simulink model "induction_machine_PeiXu_5186611"  (Simulink 8.6)
settings: Solver=ode45  StartTime=0  StopTime=25  RelTol=1e-3
libraries: aerolibutil x8
settings Model: Creator=XP  LastModifiedBy=XP
settings DataIOCC: SignalLoggingSaveFormat=Dataset
settings OptimizationCC: ExpressionDepthLimit=128
settings DebuggingCC: UnderspecifiedInitializationDetection=Simplified  MergeDetectMultiDrivingBlocksExec=error  FcnCallInpInsideContextMsg=EnableAllAsError  StateNameClashWarn=none
settings GRTTargetCC: CombineOutputUpdateFcns=on  GRTInterface=off
settings ConfigComp: CovSFcnEnable=off

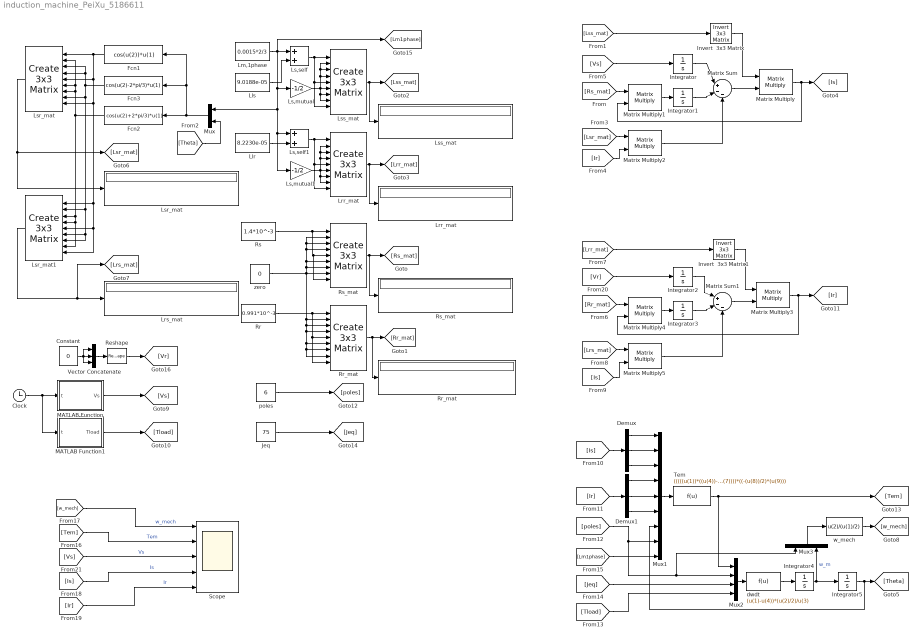
== system induction_machine_PeiXu_5186611 ==
  Clock : Clock
  Constant : Constant  Value=0
  Demux : Demux  Outputs=3
  Demux1 : Demux  Outputs=3
  Fcn1 : Fcn  Expr=cos(u(2))*u(1)
  Fcn2 : Fcn  Expr=cos(u(2)+2*pi/3)*u(1)
  Fcn3 : Fcn  Expr=cos(u(2)-2*pi/3)*u(1)
  Integrator{,1..5} (6 alike) : Integrator
  Invert  3x3 Matrix : aerolibutil/Invert  3x3 Matrix
  Invert  3x3 Matrix1 : aerolibutil/Invert  3x3 Matrix
  Jeq : Constant  Value=75
  Llr : Constant  Value=8.2230e-05
  Lls : Constant  Value=9.0188e-05
  Lm,1phase : Constant  Value=0.0015*2/3
  Lrr_mat : aerolibutil/Create 3x3 Matrix
  "Lrr_mat " : Display
  "Lrs_mat " : Display
  Ls,mutual : Gain  Gain=-1/2
  Ls,mutual1 : Gain  Gain=-1/2
  Ls,self : Sum
  Ls,self1 : Sum
  Lsr_mat : aerolibutil/Create 3x3 Matrix
  "Lsr_mat " : Display
  Lsr_mat1 : aerolibutil/Create 3x3 Matrix
  Lss_mat : aerolibutil/Create 3x3 Matrix
  "Lss_mat " : Display
  MATLAB Function : MATLAB Function  TreatAsAtomicUnit=on
  MATLAB Function1 : MATLAB Function  TreatAsAtomicUnit=on
  Matrix Sum : Sum  Inputs=|+--
  Matrix Sum1 : Sum  Inputs=|+--
  Matrix Multiply{,1..5} (6 alike) : Product  Multiplication=Matrix(*)
  Mux : Mux  Inputs=2
  Mux1 : Mux  Inputs=9
  Mux2 : Mux
  Mux3 : Mux  Inputs=2
  Reshape : Reshape  OutputDimensionality=Customize  OutputDimensions=[3,1]
  "Rr " : Constant  Value=0.991*10^-3
  Rr_mat : aerolibutil/Create 3x3 Matrix
  "Rr_mat " : Display
  Rs : Constant  Value=1.4*10^-3
  Rs_mat : aerolibutil/Create 3x3 Matrix
  "Rs_mat " : Display
  Scope : Scope  NumInputPorts=5
  Tem : Fcn  Expr=(((((u(1))*((u(4))-(0.5*(u(5)))-(0.5*(u(6)))))+((u(2))*((u(5))-(0.5*(u(4)))-(0.5*(u(6)))))+((u(3))*((u(6))-(0.5*(u(5)))-(0.5*(u(4))))))*sin(u(7)))+((sqrt(3)/2)*(((u(1))*((u(5))-(u(6))))+((u(2))*((u(6))-(u(4))))+((u(3))*((u(4))-(u(5)))))*cos(u(7))))*((-(u(8))/2)*(u(9)))
  Vector Concatenate : Concatenate  NumInputs=3
  dwdt : Fcn  Expr=(u(1)-u(4))*(u(2)/2)/u(3)
  poles : Constant  Value=6
  w_mech : Fcn  Expr=u(2)/(u(1)/2)
  "zero " : Constant  Value=0
  wires:
  Integrator/1 -> Matrix Sum/1
  Rs/1 -> Rs_mat/9, Rs_mat/5, Rs_mat/1
  "zero "/1 -> Rs_mat/4, Rs_mat/3, Rs_mat/2, Rs_mat/6, Rs_mat/7, Rr_mat/2, Rr_mat/3, Rr_mat/4, Rr_mat/6, Rr_mat/7, Rr_mat/8, Rs_mat/8
  Rs_mat/1 -> "Rs_mat "/1, [Rs_mat]
  "Rr "/1 -> Rr_mat/9, Rr_mat/5, Rr_mat/1
  Rr_mat/1 -> "Rr_mat "/1, [Rr_mat]
  Ls,self/1 -> Lss_mat/1, Lss_mat/9, Lss_mat/5
  Lls/1 -> Ls,self/2
  Ls,mutual/1 -> Lss_mat/8, Lss_mat/7, Lss_mat/4, Lss_mat/3, Lss_mat/2, Lss_mat/6
  Lss_mat/1 -> "Lss_mat "/1, [Lss_mat]
  Ls,self1/1 -> Lrr_mat/9, Lrr_mat/5, Lrr_mat/1
  Lm,1phase/1 -> [Lm1phase], Mux/1, Ls,self1/1, Ls,mutual1/1, Ls,mutual/1, Ls,self/1
  Llr/1 -> Ls,self1/2
  Ls,mutual1/1 -> Lrr_mat/8, Lrr_mat/7, Lrr_mat/4, Lrr_mat/3, Lrr_mat/2, Lrr_mat/6
  Lrr_mat/1 -> "Lrr_mat "/1, [Lrr_mat]
  [Lss_mat] -> Invert  3x3 Matrix/1
  Invert  3x3 Matrix/1 -> Matrix Multiply/1
  Matrix Sum/1 -> Matrix Multiply/2
  Matrix Multiply/1 -> [Is], Matrix Multiply1/2
  [Rs_mat] -> Matrix Multiply1/1
  Matrix Multiply1/1 -> Integrator1/1
  Integrator1/1 -> Matrix Sum/2
  Fcn2/1 -> Lsr_mat/7, Lsr_mat/6, Lsr_mat/2, Lsr_mat1/8, Lsr_mat1/4, Lsr_mat1/3
  Lsr_mat1/1 -> [Lrs_mat], "Lrs_mat "/1
  Lsr_mat/1 -> "Lsr_mat "/1, [Lsr_mat]
  Fcn1/1 -> Lsr_mat1/1, Lsr_mat1/5, Lsr_mat1/9, Lsr_mat/9, Lsr_mat/5, Lsr_mat/1
  Fcn3/1 -> Lsr_mat1/7, Lsr_mat1/6, Lsr_mat1/2, Lsr_mat/8, Lsr_mat/4, Lsr_mat/3
  [Ir] -> Matrix Multiply2/2
  [Lsr_mat] -> Matrix Multiply2/1
  Matrix Multiply2/1 -> Matrix Sum/3
  [Vs] -> Integrator/1
  Integrator2/1 -> Matrix Sum1/1
  [Lrr_mat] -> Invert  3x3 Matrix1/1
  Invert  3x3 Matrix1/1 -> Matrix Multiply3/1
  Matrix Sum1/1 -> Matrix Multiply3/2
  Matrix Multiply3/1 -> [Ir], Matrix Multiply4/2
  [Rr_mat] -> Matrix Multiply4/1
  Matrix Multiply4/1 -> Integrator3/1
  Integrator3/1 -> Matrix Sum1/2
  [Is] -> Matrix Multiply5/2
  [Lrs_mat] -> Matrix Multiply5/1
  Matrix Multiply5/1 -> Matrix Sum1/3
  [Vr] -> Integrator2/1
  [Is] -> Demux/1
  [Ir] -> Demux1/1
  Demux/1 -> Mux1/1
  Demux/2 -> Mux1/2
  Demux/3 -> Mux1/3
  Demux1/1 -> Mux1/4
  Demux1/2 -> Mux1/5
  Demux1/3 -> Mux1/6
  poles/1 -> [poles]
  Mux1/1 -> Tem/1
  Tem/1 -> [Tem], Mux2/1
  Jeq/1 -> [Jeq]
  Integrator4/1 -> Integrator5/1, Mux3/2  "w_m"
  Integrator5/1 -> Mux1/7, [Theta]
  Mux2/1 -> dwdt/1
  [Jeq] -> Mux2/3
  [Tload] -> Mux2/4
  dwdt/1 -> Integrator4/1
  [Tem] -> Scope/2  "Tem"
  [Is] -> Scope/4  "Is"
  [Lm1phase] -> Mux1/9
  MATLAB Function/1(Vs) -> [Vs]
  [Theta] -> Mux/2
  Mux/1 -> Fcn3/1, Fcn1/1, Fcn2/1
  Clock/1 -> MATLAB Function1/1(t), MATLAB Function/1(t)
  MATLAB Function1/1(Tload) -> [Tload]
  [poles] -> Mux1/8, Mux3/1, Mux2/2
  Mux3/1 -> w_mech/1
  w_mech/1 -> [w_mech]
  [Vs] -> Scope/3  "Vs"
  Reshape/1 -> [Vr]
  Vector Concatenate/1 -> Reshape/1
  Constant/1 -> Vector Concatenate/3, Vector Concatenate/1, Vector Concatenate/2
  [Ir] -> Scope/5  "Ir"
  [w_mech] -> Scope/1  "w_mech"

== matlab function MATLAB Function1 ==
  data: t input double; Tload output double
function Tload = Tload_func(t)

starting_time = 15;
 
if t < starting_time
    Tload = 0;
elseif t < starting_time + 5
    Tload = 1.6544*10^4;
else
    Tload = 0.75*1.6544*10^4;
end

== matlab function MATLAB Function ==
  data: t input double; Vs output double
function Vs = Vs_func(t)

V_rated_phase = 575/sqrt(3); % V

starting_time = 3;
full_voltage_time = 5;

if t < starting_time
    Vs = [0 0 0]';
elseif t < full_voltage_time
    rate = (t-starting_time)/(full_voltage_time-starting_time);
    Vs = [rate * V_rated_phase * sqrt(2) * cos(120*pi*(t-starting_time));...
        rate * V_rated_phase * sqrt(2) * cos(120*pi*(t-starting_time) - 2*pi/3);...
        rate * V_rated_phase * sqrt(2) * cos(120*pi*(t-starting_time) + 2*pi/3)];
else
    Vs =[V_rated_phase * sqrt(2) * cos(120*pi*(t-starting_time));...
        V_rated_phase * sqrt(2) * cos(120*pi*(t-starting_time) - 2*pi/3);...
        V_rated_phase * sqrt(2) * cos(120*pi*(t-starting_time) + 2*pi/3)];
end
